simulink model "onlySF1"  (Simulink 9.2)
settings: Solver=VariableStepAuto  StartTime=0.0  StopTime=60  RelTol=1e-3
settings Model: Creator=jinwooro  LastModifiedBy=jinwooro
settings DataIOCC: LimitDataPoints=off  SaveFormat=Dataset  SignalLoggingSaveFormat=Dataset
settings OptimizationCC: LifeSpan=auto
settings DebuggingCC: UnderspecifiedInitializationDetection=Simplified  MergeDetectMultiDrivingBlocksExec=error  FcnCallInpInsideContextMsg=error  StateNameClashWarn=none  SFUnexpectedBacktrackingDiag=error  SFNoUnconditionalDefaultTransitionDiag=error  SFExecutionAtInitializationDiag=warning
settings HardwareCC: ProdBitPerPointer=64  ProdBitPerSizeT=64  ProdBitPerPtrDiffT=64  ProdLargestAtomicFloat=Float  ProdIntDivRoundTo=Zero  ProdEndianess=LittleEndian  ProdWordSize=64  ProdHWDeviceType=Intel->x86-64 (Windows64)
settings ModelReferenceCC: PropagateSignalLabelsOutOfModel=on
settings SFSimCC: SimUseLocalCustomCode=on
settings RTWCC: RTWUseLocalCustomCode=on
settings CodeAppCC: StateflowObjectComments=off
settings GRTTargetCC: TargetLangStandard=C99 (ISO)  GeneratePreprocessorConditionals=Use local settings  CombineOutputUpdateFcns=on  GRTInterface=off
settings ConfigComp: CovMetricSettings=dwe  CovHtmlReporting=off  CovSaveCumulativeToWorkspaceVar=off  CovSaveSingleToWorkspaceVar=off  CovExternalEMLEnable=on

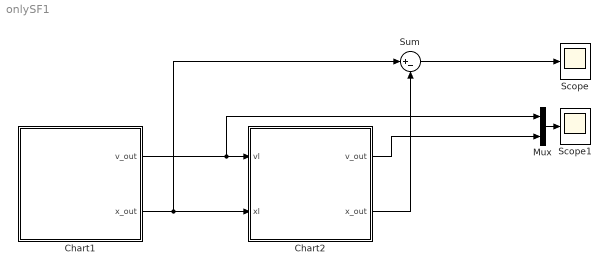
== system onlySF1 ==
  Chart1 : Stateflow chart  TreatAsAtomicUnit=on
  Chart2 : Stateflow chart  TreatAsAtomicUnit=on
  Mux : Mux  Inputs=2
  Scope : Scope
  Scope1 : Scope
  Sum : Sum  Inputs=|+-
  wires:
  Chart1/1(v_out) -> Mux/1, Chart2/1(vl)
  Chart1/2(x_out) -> Sum/1, Chart2/2(xl)
  Sum/1 -> Scope/1
  Chart2/2(x_out) -> Sum/2
  Mux/1 -> Scope1/1
  Chart2/1(v_out) -> Mux/2

== stateflow chart Chart2 ==
  settings: updateMethod=CONTINUOUS
  state LocB
    du:
    v_dot = 0;
    x_dot = 0;
    v_out = v;
    x_out = x;
  state LocA
    du:
    v_dot = 0.9 * (vl-v);
    x_dot = v;
    v_out = v;
    x_out = x;
  (default) -> LocA : {x = -25;
      | v = 0;}
  LocA -> LocB : [power(xl - x, 0.5) < 0]{v = 0;}
  data: v_out output double; vl input double; x_out output double; v local double; x local double; xl input double
  data vl settings: updateMethod=SF_CONTINUOUS_TIME_DATA
  data v settings: updateMethod=SF_CONTINUOUS_TIME_DATA
  data x settings: updateMethod=SF_CONTINUOUS_TIME_DATA
  data xl settings: updateMethod=SF_CONTINUOUS_TIME_DATA

== stateflow chart Chart1 ==
  settings: updateMethod=CONTINUOUS
  state LocB
    en:
    v = 25;
    du:
    v_dot = -2;
    x_dot = v;
    v_out = v;
    x_out = x;
  state LocA
    du:
    v_dot = 2;
    x_dot = v;
    v_out = v;
    x_out = x;
  (default) -> LocA : {x = 0;
      | v= 0;}
  LocA -> LocB : [v >= 25]
  LocB -> LocA : [v <= 13]
  data: v_out output double; x local double; x_out output double; v local double
  data x settings: updateMethod=SF_CONTINUOUS_TIME_DATA
  data v settings: updateMethod=SF_CONTINUOUS_TIME_DATA
